simulink model "dspsdadc2"  (Simulink 7.4)
settings: Solver=ode23  SolverMode=SingleTasking  StartTime=0.0  StopTime=120/8000  FixedStep=1/512000  RelTol=1e-3  AbsTol=1e-6
libraries: dspmlti4 x3, dsparch4 x1, simulink x1, dspobslib x1
settings Model: Creator=don  LastModifiedBy=Dick  ExtModeTrigMode=oneshot  ExtModeArmWhenConnect=off
settings DataIOCC: LimitDataPoints=off  SaveOutput=off  SignalLoggingName=sigsOut
settings OptimizationCC: BlockReduction=off  BooleanDataType=off  InitFltsAndDblsToZero=on
settings DebuggingCC: SaveWithParameterizedLinksMsg=none  SignalResolutionControl=TryResolveAllWithWarning  SolverPrmCheckMsg=none  MultiTaskDSMMsg=warning  MultiTaskCondExecSysMsg=none  IntegerOverflowMsg=none  StrictBusMsg=None
settings HardwareCC: TargetUnknown=on
settings RTWCC: IncludeERTFirstTime=on
settings GRTTargetCC: TargetFcnLib=ansi_tfl_tmw.mat

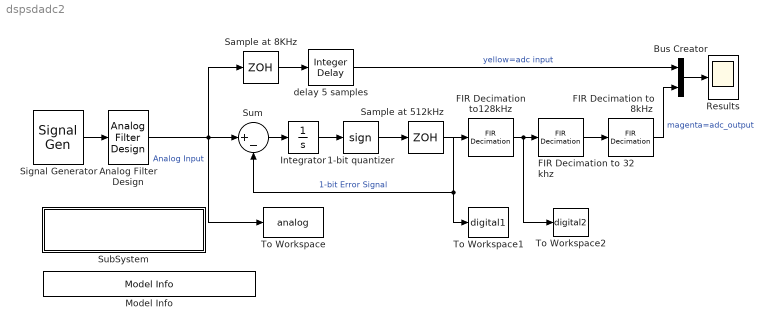
== system dspsdadc2 ==
  1-bit quantizer : Signum
  Analog Filter Design : dsparch4/Analog Filter Design  method=Butterworth  filttype=Lowpass  N=5  Wlo=2*pi*400  Whi=80  Rp=2  Rs=40
  Bus Creator : BusCreator  Inputs=2
  FIR Decimation to 32 khz : dspmlti4/FIR Decimation  DialogController=dspdialog.FIRDecimation  DialogControllerArgs=DataTag0  h=fir1(31, 0.15)  D=4  filtStruct=Direct form  framing=Maintain input frame size  outputBufInitCond=0  roundingMode=Floor  overflowMode=off  FilterSource=Specify via dialog  FilterObject=Hm_firdecim
  FIR Decimation to 8kHz : dspmlti4/FIR Decimation  DialogController=dspdialog.FIRDecimation  DialogControllerArgs=DataTag1  h=fir1(31, 0.15)  D=4  filtStruct=Direct form  framing=Maintain input frame size  outputBufInitCond=0  roundingMode=Floor  overflowMode=off  FilterSource=Specify via dialog  FilterObject=Hm_firdecim
  FIR Decimation to128kHz : dspmlti4/FIR Decimation  DialogController=dspdialog.FIRDecimation  DialogControllerArgs=DataTag2  h=fir1(31, 0.15)  D=4  filtStruct=Direct form  framing=Maintain input frame size  outputBufInitCond=0  roundingMode=Floor  overflowMode=off  FilterSource=Specify via dialog  FilterObject=Hm_firdecim
  Integrator : Integrator
  Model Info : simulink/Model-Wide Utilities/Model Info  SystemSampleTime=-1  InitialBlockCM=none  BlockCM=none  Frame=on  DisplayStringWithTags=Copywrite 2005-2010 The MathWorks, Inc.  HorizontalTextAlignment=Center  LeftAlignmentValue=0.5  SourceBlockDiagram=dspsdadc2  TagMaxNumber=20
  Results : Scope
      settings: TimeRange=0.015  YMin=-1  YMax=1  DataFormat=Array
  Sample at 512kHz : ZeroOrderHold  SampleTime=1/512000
  Sample at 8KHz : ZeroOrderHold  SampleTime=1/8000
  Signal Generator : SignalGenerator  WaveForm=square  Amplitude=0.75  Frequency=80
  SubSystem : Subsystem
      settings: OpenFcn=plot_signal
      mask Display: disp('Plot signals using MATLAB.\n Note the minimum time step size.')
  Sum : Sum  Inputs=|+-  OutDataType=sfix(16)  OutScaling=2^0  SaturateOnIntegerOverflow=on  InputSameDT=on  OutDataTypeStr=Inherit: Same as first input
  To Workspace : ToWorkspace  VariableName=analog  SampleTime=-1  SaveFormat=Structure With Time
  To Workspace1 : ToWorkspace  VariableName=digital1  SampleTime=-1  SaveFormat=Structure With Time
  To Workspace2 : ToWorkspace  VariableName=digital2  SampleTime=-1  SaveFormat=Structure With Time
  delay 5 samples : dspobslib/Integer Delay  delay=5  ic=0  reset_popup=None
  wires:
  FIR Decimation to 32 khz/1 -> FIR Decimation to 8kHz/1
  FIR Decimation to 8kHz/1 -> Bus Creator/2  "magenta=adc_output"
  Analog Filter Design/1 -> Sum/1, To Workspace/1, Sample at 8KHz/1  "Analog Input"
  Signal Generator/1 -> Analog Filter Design/1
  1-bit quantizer/1 -> Sample at 512kHz/1
  Sample at 512kHz/1 -> FIR Decimation to128kHz/1, Sum/2, To Workspace1/1  "1-bit Error Signal"
  Sum/1 -> Integrator/1
  FIR Decimation to128kHz/1 -> FIR Decimation to 32 khz/1, To Workspace2/1
  Integrator/1 -> 1-bit quantizer/1
  Bus Creator/1 -> Results/1
  Sample at 8KHz/1 -> delay 5 samples/1
  delay 5 samples/1 -> Bus Creator/1  "yellow=adc input"

== system dspsdadc2/SubSystem ==
